simulink subsystem "Power_Stage"  (R2022a)
settings: Solver=VariableStepAuto  StartTime=0.0  StopTime=10.0  RelTol=1e-3
libraries: spsMosfetLib x4, spsSeriesRLCBranchLib x3, spsCurrentMeasurementLib x2, spsVoltageMeasurementLib x1, spsPWMGeneratorDCDCLib x1, spspowerguiLib x1
settings Model: Creator=Blank  LastModifiedBy=Blank

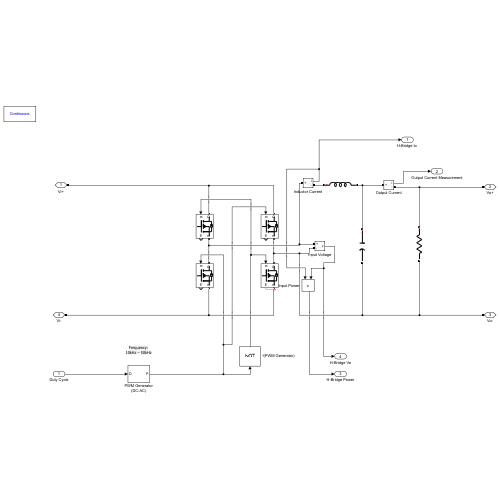
[thumbnail: Simulink's stored preview of the top-level diagram]
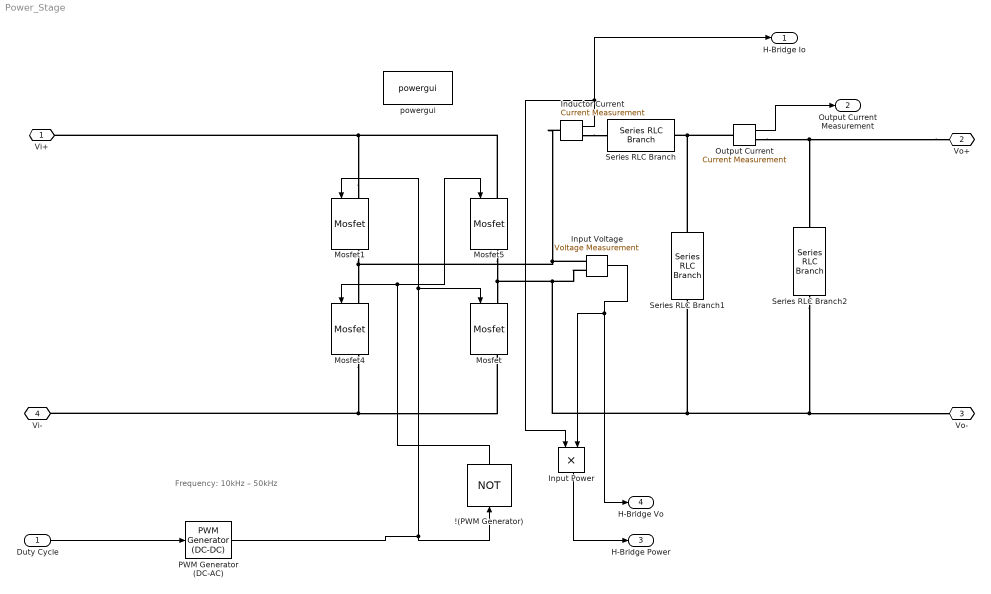
== system Power_Stage ==
  note: Frequency:
      | 10kHz – 50kHz
  Duty Cycle : Inport
  !(PWM Generator) : Logic  Operator=NOT  AllPortsSameDT=off  OutDataTypeStr=boolean
  Inductor Current : spsCurrentMeasurementLib/Current Measurement  PhasorSimulation=off  OutputType=Complex  PSBequivalent=0
  Input Power : Product
  Input Voltage : spsVoltageMeasurementLib/Voltage Measurement  PhasorSimulation=off  OutputType=Complex  PSBequivalent=0
  Mosfet{,1,4..5} (4 alike) : spsMosfetLib/Mosfet  Ron=0.1  Lon=0  Rd=0.01  Vfd=0  IC=0  Rs=1e5  Cs=inf  Measurements=on
  Output Current : spsCurrentMeasurementLib/Current Measurement  PhasorSimulation=off  OutputType=Complex  PSBequivalent=0
  PWM Generator (DC-AC) : spsPWMGeneratorDCDCLib/PWM Generator (DC-DC)  Fsw=30e3  Ts=0
  Series RLC Branch : spsSeriesRLCBranchLib/Series RLC Branch  LConnTagsString=__new0  RConnTagsString=__new0  BranchType=L  Resistance=1  Inductance=2.5e-3  SetiL0=off  InitialCurrent=0  Capacitance=1e-6  Setx0=off  InitialVoltage=0  Measurements=Branch current
  Series RLC Branch1 : spsSeriesRLCBranchLib/Series RLC Branch  LConnTagsString=__new0  RConnTagsString=__new0  BranchType=C  Resistance=1  Inductance=1e-3  SetiL0=off  InitialCurrent=0  Capacitance=2e-6  Setx0=off  InitialVoltage=0  Measurements=None
  Series RLC Branch2 : spsSeriesRLCBranchLib/Series RLC Branch  LConnTagsString=__new0  RConnTagsString=__new0  BranchType=R  Resistance=2.2  Inductance=1e-3  SetiL0=off  InitialCurrent=0  Capacitance=1e-6  Setx0=off  InitialVoltage=0  Measurements=None
  powergui : spspowerguiLib/powergui  Priority=1  SimulationMode=Continuous  SampleTime=50e-6  frequency=60  Iterations=50  frequencyindice=0  Pbase=100e6  ErrMax=1e-4  UnitsV=kV  UnitsW=MW  buscounter=0  FunctionMessages=off  echomessages=off  EnableUseOfTLC=off  CurrentSourceSwitches=off  DisableSnubberDevices=off  DisableRonSwitches=off  DisableVfSwitches=off  DisplayEquations=off  AutomaticDiscreteSolvers=off  SolverType=Tustin/Backward Euler (TBE)  Interpol=off  ExternalGateDelay=off  methode=off  Ts=100  x0status=blocks  SPID=on  SwTol=0  HookPort=off  NonlinearTolerance=1e-4  nMaxIteration=100  ContinueOnMaxIteration=off  RestoreLinks=warning  ResistiveCurrentMeasurement=off  Frange=[0:2:500]  Ylog=off  Xlog=on  ShowGrid=off  save=off  variable=ZData  structure=0  ZoomFFT=off  StartTime=0.0  cycles=1  DisplayStyle=1  fundamental=60  FreqAxis=off  MaxFrequency=1000  frequencyindicesteady=1  RmsSteady=1  display=off
  Vi+ : PMIOPort  Side=Left
  Vo+ : PMIOPort  Port=2  Side=Right
  Vo- : PMIOPort  Port=3  Side=Right
  Vi- : PMIOPort  Port=4  Side=Left
  "H-Bridge Io " : Outport
  Output Current Measurement : Outport  Port=2
  H-Bridge Power : Outport  Port=3
  H-Bridge Vo : Outport  Port=4
  wires:
  Duty Cycle/1 -> PWM Generator (DC-AC)/1
  Input Voltage/1 -> H-Bridge Vo/1, Input Power/2
  Inductor Current/1 -> "H-Bridge Io "/1, Input Power/1
  Output Current/1 -> Output Current Measurement/1
  PWM Generator (DC-AC)/1 -> Mosfet1/1, Mosfet/1, !(PWM Generator)/1
  Input Power/1 -> H-Bridge Power/1
  !(PWM Generator)/1 -> Mosfet4/1, Mosfet5/1
  connections:
  Input Voltage/LConn1 -- Mosfet1/RConn1 -- Mosfet4/LConn1 -- Inductor Current/LConn1
  Series RLC Branch2/RConn1 -- Mosfet5/RConn1 -- Mosfet/LConn1 -- Input Voltage/LConn2 -- Series RLC Branch1/RConn1 -- Vo-/RConn1
  Series RLC Branch/RConn1 -- Series RLC Branch1/LConn1 -- Output Current/LConn1
  Mosfet/RConn1 -- Vi-/RConn1 -- Mosfet4/RConn1
  Vo+/RConn1 -- Series RLC Branch2/LConn1 -- Output Current/RConn1
  Mosfet1/LConn1 -- Vi+/RConn1 -- Mosfet5/LConn1
  Inductor Current/RConn1 -- Series RLC Branch/LConn1
